simulink model "test"  (Simulink 7.8)
settings: Solver=ode1  StartTime=0.0  StopTime=inf  FixedStep=0.002  RelTol=1e-3
undefined symbols (not defined in the file or in its folder): HIL, qc_get_step_size
libraries: quarc_library x3
settings Model: Creator=frouss7  LastModifiedBy=frouss7  SimulationMode=external  ExtModeTrigDuration=5000
settings SolverCC: PositivePriorityOrder=on
settings RTWCC: SystemTargetFile=quarc_win64.tlc  TemplateMakefile=quarc_default_tmf  Description=QUARC Win64 Target  ProcessScript=quarc_win64_make_rtw_hook
settings STFCustomTargetCC: TargetPreCompLibLocation=C:\PROGRA~3\QUARC\lib\2011b\win64\release  SystemTargetFile=quarc_win64.tlc
settings GRTTargetCC: TargetPreCompLibLocation=C:\PROGRA~3\QUARC\lib\2011b\win64\release  ParMdlRefBuildCompliant=off  CompOptLevelCompliant=off  ConcurrentExecutionCompliant=off  MatFileLogging=off  ExtMode=on  ExtModeMexFile=quarc_comm

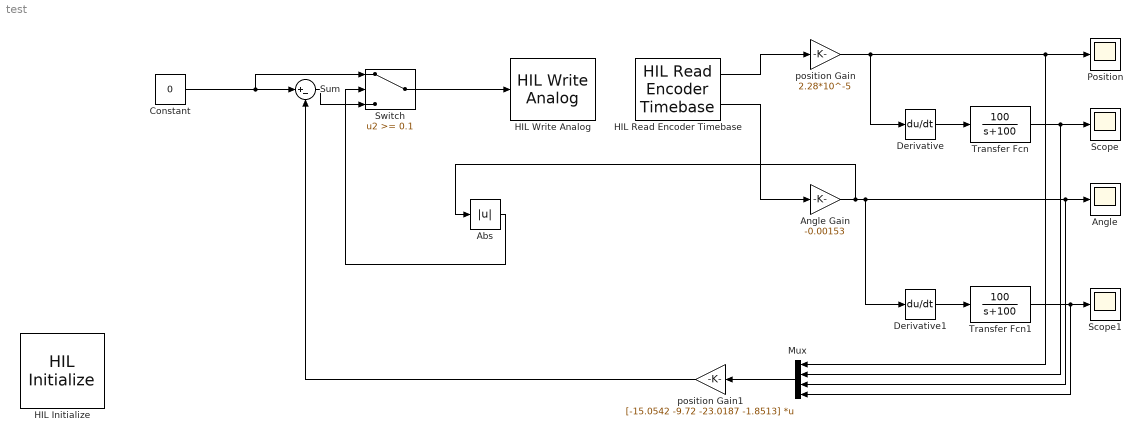
== system test ==
  Abs : Abs
  Angle : Scope
      settings: YMin=-0.6  YMax=0.6
  Angle Gain : Gain  Gain=-0.00153
  Constant : Constant  Value=0
  Derivative : Derivative
  Derivative1 : Derivative
  HIL Initialize : quarc_library/Data Acquisition/Generic/Configuration/HIL Initialize  Priority=-99  object_name=HIL-1  board_type=q4  board_number=0  exclusive=off  active=off  hardware_clocks=[0:1]  clock_modes=[0 0]  initial_clock_frequencies=[]  set_clock_params_at_start=on  set_clock_params_at_switch_in=off  set_clock_frequencies_at_start=off  set_clock_frequencies_at_switch_in=off  analog_input_channels=[0:3]  analog_input_maximums=10  analog_input_minimums=-10  set_analog_input_params_at_start=off  set_analog_input_params_at_switch_in=off  analog_output_channels=[0:3]  analog_output_maximums=[10]  analog_output_minimums=[-10]  initial_analog_outputs=[0]  final_analog_outputs=[0]  watchdog_analog_outputs=0  set_analog_output_params_at_start=on  set_analog_output_params_at_switch_in=off  set_analog_outputs_at_start=on  set_analog_outputs_at_switch_in=off  set_analog_outputs_at_terminate=on  set_analog_outputs_at_switch_out=off  set_analog_outputs_on_watchdog=off  digital_input_channels=[]  digital_output_channels=[]  digital_output_configuration=[]  initial_digital_outputs=[1]  final_digital_outputs=[1]  watchdog_digital_outputs=[2]  set_digital_output_params_at_start=off  set_digital_output_params_at_switch_in=off  set_digital_outputs_at_start=on  set_digital_outputs_at_switch_in=off  set_digital_outputs_at_terminate=on  set_digital_outputs_at_switch_out=off  set_digital_outputs_on_watchdog=off  encoder_channels=[0:3]  quadrature=[4]  encoder_filter_frequency=(1/60e-9)/1  initial_encoder_counts=[0]  set_encoder_params_at_start=on  set_encoder_params_at_switch_in=off  set_encoder_counts_at_start=on  set_encoder_counts_at_switch_in=off  pwm_channels=[]  pwm_modes=[0]  pwm_frequency=(1/60e-9)/1024  pwm_configuration=[]  pwm_alignment=[]  pwm_polarity=[]  pwm_leading_deadband=[]  pwm_trailing_deadband=[]  initial_pwm_outputs=[0]  final_pwm_outputs=[0]  watchdog_pwm_outputs=[]  set_pwm_params_at_start=on  set_pwm_params_at_switch_in=off  set_pwm_outputs_at_start=on  set_pwm_outputs_at_switch_in=off  set_pwm_outputs_at_terminate=on  set_pwm_outputs_at_switch_out=off  set_pwm_outputs_on_watchdog=off  other_output_channels=[]  initial_other_outputs=[]  final_other_outputs=[]  watchdog_other_outputs=[]  set_other_outputs_at_start=off  set_other_outputs_at_switch_in=off  set_other_outputs_at_terminate=off  set_other_outputs_at_switch_out=off  set_other_outputs_on_watchdog=off
  HIL Read Encoder Timebase : quarc_library/Data Acquisition/Generic/Timebases/HIL Read Encoder Timebase  object_name=HIL-1  clock=0  channels=[0 1]  samples_in_buffer=max(ceil(1/qc_get_step_size), 1)  active=on  vector_output=off  data_type_mode=Inherit via back propagation  data_type=double
  HIL Write Analog : quarc_library/Data Acquisition/Generic/Immediate I//O/HIL Write Analog  object_name=HIL-1  channels=0  sample_time=-1  active=off  vector_input=off
  Mux : Mux
  Position : Scope
      settings: TimeRange=0.6069767441860465  YMin=-15  YMax=15
  Scope : Scope
      settings: SaveName=ScopeData2
  Scope1 : Scope
      settings: SaveName=ScopeData3
  Sum : Sum  Inputs=|+-
  Switch : Switch  Threshold=0.1
  Transfer Fcn : TransferFcn  Numerator=[100]  Denominator=[1 100]
  Transfer Fcn1 : TransferFcn  Numerator=[100]  Denominator=[1 100]
  position Gain : Gain  Gain=2.28*10^-5
  position Gain1 : Gain  Gain=[-15.0542 -9.72 -23.0187 -1.8513]  Multiplication=Matrix(K*u) (u vector)
  wires:
  position Gain/1 -> Derivative/1, Mux/1, Position/1
  Angle Gain/1 -> Derivative1/1, Angle/1, Mux/3, Abs/1
  Derivative/1 -> Transfer Fcn/1
  Transfer Fcn/1 -> Scope/1, Mux/2
  Derivative1/1 -> Transfer Fcn1/1
  Transfer Fcn1/1 -> Scope1/1, Mux/4
  Mux/1 -> position Gain1/1
  position Gain1/1 -> Sum/2
  Constant/1 -> Sum/1, Switch/1
  HIL Read Encoder Timebase/1 -> position Gain/1
  HIL Read Encoder Timebase/2 -> Angle Gain/1
  Sum/1 -> Switch/3
  Abs/1 -> Switch/2
  Switch/1 -> HIL Write Analog/1
